simulink model "up2Control"  (R2017b)
settings: Solver=FixedStepAuto  StartTime=0.0  StopTime=15  FixedStep=1e-3  RelTol=1e-3
values from neighbouring files (symbols this model uses):
  Klqr3 = designLQR(A2, B2, diag([900,0,100,0]), 1)    [calcSystem.m]
settings Model: Creator=Haotian  LastModifiedBy=Haotian

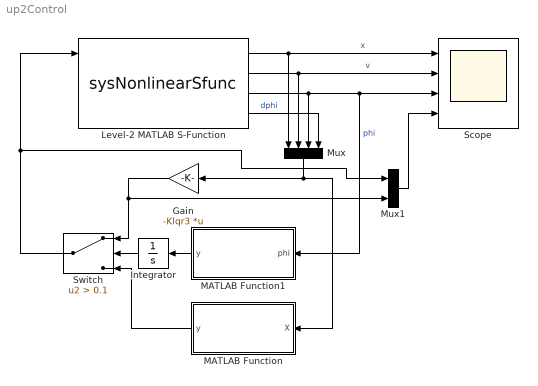
== system up2Control ==
  Gain : Gain  Gain=-Klqr3  Multiplication=Matrix(K*u)
  Integrator : Integrator
  Level-2 MATLAB S-Function : M-S-Function  FunctionName=sysNonlinearSfunc  Parameters=Mc, Mg, b, l, I, init_phi, useAcc  mask(S-function: sysNonlinearSfunc){Mc=1.096, Mg=0.109, b=0.1, l=0.25, I=0.0034, init_phi=pi - 0.01, useAcc=on}
      mask prompts: Mc "小车质量"; Mg "摆杆质量"; b "小车摩擦系数"; l "摆杆转动轴心到杆质心的长度"; I "摆杆惯量"; init_phi "初始垂直夹角"; useAcc "使用加速度作为输入"
      mask help: 一阶倒立摆非线性模型。
      mask Display:
      | fprintf('一阶倒立摆\n\nM=%.3f m=%.3f\nb=%.3f l=%.3f\nI=%.3f phi0=%.2f\n\nX=[x dx phi dphi]', Mc, Mg, b, l, I, init_phi);
      | if(useAcc)
      |     port_label('input', 1, 'a');
      | else
      |     port_label('input', 1, 'F');
      | end
      | port_label('input', 2, 'setX');
      | port_label('input', 3, 'devX');
      | 
      | port_label('output', 1, 'x');
      | port_label('output', 2, 'v');
      | port_label('output', 3, '\phi','texmode','on');
      | port_label('output', 4, 'd\phi','texmode','on');
  MATLAB Function : MATLAB Function  TreatAsAtomicUnit=on
  MATLAB Function1 : MATLAB Function  TreatAsAtomicUnit=on
  Mux : Mux
  Mux1 : Mux  Inputs=2
  Scope : Scope  NumInputPorts=4
  Switch : Switch  Criteria=u2 > Threshold  Threshold=0.1
  wires:
  MATLAB Function1/1(y) -> Integrator/1
  Mux/1 -> MATLAB Function/1(X), Gain/1
  Level-2 MATLAB S-Function/2 -> Scope/2, Mux/2  "v"
  MATLAB Function/1(y) -> Switch/3
  Level-2 MATLAB S-Function/4 -> Mux/4  "dphi"
  Level-2 MATLAB S-Function/3 -> MATLAB Function1/1(phi), Scope/3, Mux/3  "phi"
  Level-2 MATLAB S-Function/1 -> Mux/1, Scope/1  "x"
  Gain/1 -> Switch/1, Mux1/2
  Switch/1 -> Mux1/1, Level-2 MATLAB S-Function/1
  Integrator/1 -> Switch/2
  Mux1/1 -> Scope/4

== matlab function up2Control/MATLAB Function1 ==
  data: phi input; y output
function y = switchControl(phi)
if(abs(phi) < pi/7.57)
    y = 1;
else
    y = 0;
end

== matlab function up2Control/MATLAB Function ==
  data: X input; y output
function y = swingUp(X)
x = X(1);
phi = X(3);
dphi = X(4);
eps = 1e-5;
m = 0.109;
l = 0.25;
I = 1/3*m*l^2;% 0.0034;
g = 9.80;
umax = 0.1 * g;
if(abs(cos(phi)) < eps || abs(dphi) < eps)
   y = 0; 
else
    y = ( - sign((1/2*(I + m * l^2)*dphi^2+m*g*l*(cos(phi)-1))*dphi*cos(phi))) * umax;
    if(sign(y * x) > 0)
        y = 0;
    end
end
